simulink model "a3flugzeugSimpleBlock"  (R2020b)
settings: Solver=VariableStepAuto  StartTime=0.0  StopTime=12  RelTol=1e-3
settings Model: Creator=ReichlJakob  LastModifiedBy=jakob
settings DataIOCC: ReturnWorkspaceOutputs=off
settings DebuggingCC: ArithmeticOperatorsInVariantConditions=warning
settings SFSimCC: SimUseLocalCustomCode=off  CustomCodeUndefinedFunction=UseInterfaceOnly
settings RTWCC: RTWUseLocalCustomCode=off

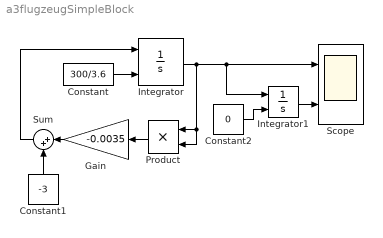
== system a3flugzeugSimpleBlock ==
  Constant : Constant  Value=300/3.6
  Constant1 : Constant  Value=-3
  Constant2 : Constant  Value=0
  Gain : Gain  Gain=-0.0035
  Integrator : Integrator  InitialConditionSource=external
  Integrator1 : Integrator  InitialConditionSource=external
  Product : Product
  Scope : Scope  NumInputPorts=2
  Sum : Sum  Inputs=|++
  wires:
  Constant/1 -> Integrator/2
  Integrator/1 -> Product/2, Product/1, Scope/1, Integrator1/1
  Product/1 -> Gain/1
  Sum/1 -> Integrator/1
  Gain/1 -> Sum/1
  Constant1/1 -> Sum/2
  Integrator1/1 -> Scope/2
  Constant2/1 -> Integrator1/2
